simulink model "lab2_part2"  (R2022a)
settings: Solver=VariableStepAuto  StartTime=0.0  StopTime=10.0  RelTol=1e-3
settings Model: Creator=minkyu3  LastModifiedBy=minkyu3

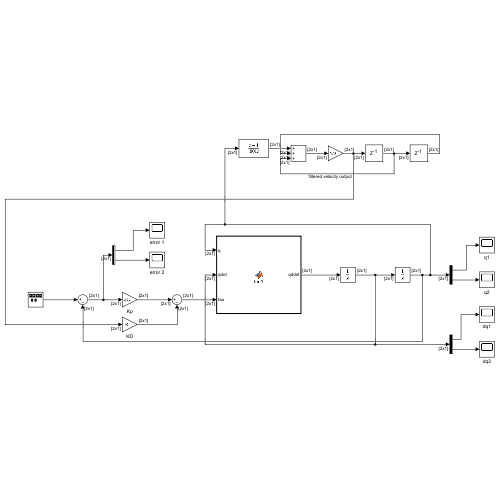
[thumbnail: Simulink's stored preview of the top-level diagram]
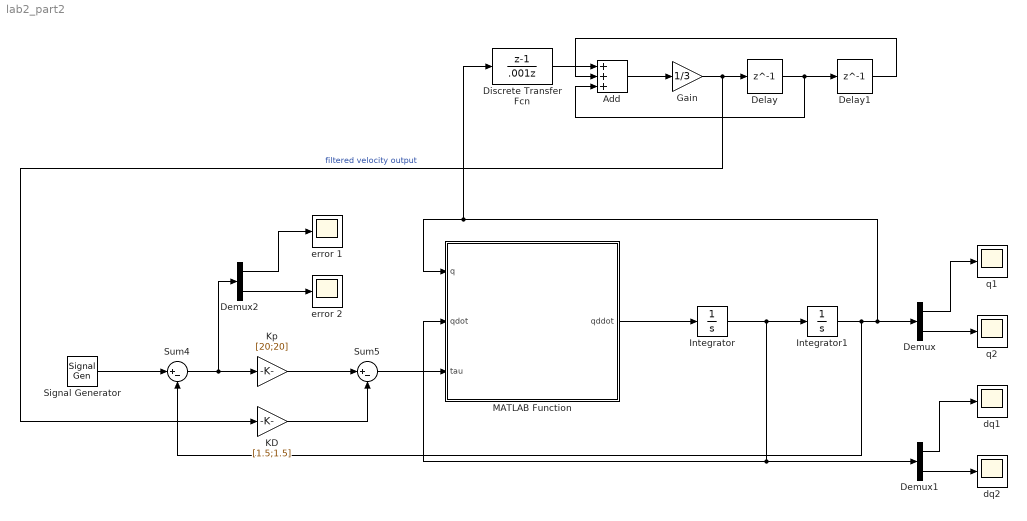
== system lab2_part2 ==
  Add : Sum  Inputs=+++
  Delay : Delay  DelayLength=1  SampleTime=0.001
  Delay1 : Delay  DelayLength=1  SampleTime=0.001
  Demux : Demux  Outputs=2
  Demux1 : Demux  Outputs=2
  Demux2 : Demux  Outputs=2
  Discrete Transfer Fcn : DiscreteTransferFcn  Numerator=[1 -1]  Denominator=[.001 0]  SampleTime=0.001
  Gain : Gain  Gain=1/3
  Integrator : Integrator  InitialCondition=[0;0]
  Integrator1 : Integrator  InitialCondition=[0;0]
  KD : Gain  Gain=[1.5;1.5]
  Kp : Gain  Gain=[20;20]
  MATLAB Function : MATLAB Function  TreatAsAtomicUnit=on
  Signal Generator : SignalGenerator  WaveForm=square  Amplitude=0.1  Frequency=0.25
  Sum4 : Sum  Inputs=|+-
  Sum5 : Sum  Inputs=|+-
  dq1 : Scope
  dq2 : Scope
  error 1 : Scope
  error 2 : Scope
  q1 : Scope
  q2 : Scope
  wires:
  MATLAB Function/1(qddot) -> Integrator/1
  Integrator/1 -> Demux1/1, MATLAB Function/2(qdot), Integrator1/1
  Integrator1/1 -> Discrete Transfer Fcn/1, MATLAB Function/1(q), Demux/1, Sum4/2
  Demux/2 -> q2/1
  Demux/1 -> q1/1
  Demux1/2 -> dq2/1
  Demux1/1 -> dq1/1
  Discrete Transfer Fcn/1 -> Add/1
  Add/1 -> Gain/1
  Gain/1 -> KD/1, Delay/1  "filtered velocity output"
  Delay/1 -> Add/3, Delay1/1
  Delay1/1 -> Add/2
  Signal Generator/1 -> Sum4/1
  Sum4/1 -> Demux2/1, Kp/1
  Kp/1 -> Sum5/1
  KD/1 -> Sum5/2
  Sum5/1 -> MATLAB Function/3(tau)
  Demux2/2 -> error 2/1
  Demux2/1 -> error 1/1

== matlab function lab2_part2/MATLAB Function ==
  data: q input; qddot output; qdot input; tau input
function qddot = fcn1(q, qdot, tau)

g = 9.81;

p = [0.03; 0.0128; 0.0076; 0.0753; 0.0298];
D = [p(1), -p(3)*sin(q(2)-q(1)); -p(3)*sin(q(2)-q(1)), p(2)];
C = [0, -p(3)*cos(q(2)-q(1))*qdot(2); p(3)*cos(q(2)-q(1))*qdot(1), 0];
G = [-p(4)*g*sin(q(1)); -p(5)*g*cos(q(2))];

qddot = D\tau - D\C*qdot - D\G;
